simulink model "Human_Driver"  (R2024b)
settings: Solver=ode1  StartTime=0.0  StopTime=inf  FixedStep=0.01  RelTol=1e-3
libraries: rFproPhysicsLib x13
settings Model: ParamWorkspaceSource=ReferencedWorkspace  TunableVars=LOCAL_PORT_RECV,REMOTE_PORT_RECV,gCGHeight,gFrontTrack,gFrontWheelRadius,gLeftWheelBase,gRearTrack,gRearWheelRadius,gRightWheelBase  TunableVarsStorageClass=Auto,Auto,Auto,Auto,Auto,Auto,Auto,Auto,Auto  TunableVarsTypeQualifier=,,,,,,,,  Creator=enewton  LastModifiedBy=Saian
settings SolverCC: AlgebraicLoopSolver=TrustRegion
settings DataIOCC: LimitDataPoints=on  SaveFormat=Array  SignalLoggingSaveFormat=ModelDataLogs  SaveOutput=off  SignalLogging=off  DSMLogging=off  SaveTime=off  ReturnWorkspaceOutputs=off
settings OptimizationCC: BlockReduction=off  ConditionallyExecuteInputs=off  OptimizeBlockIOStorage=off  BufferReuse=off  GlobalBufferReuse=off  ExpressionFolding=off  ExpressionDepthLimit=2147483647  LocalBlockOutputs=off  LifeSpan=inf  OptimizeDataStoreBuffers=off  BusAssignmentInplaceUpdate=off
settings DebuggingCC: UnderspecifiedInitializationDetection=Classic  MergeDetectMultiDrivingBlocksExec=none  SolverPrmCheckMsg=warning  FcnCallInpInsideContextMsg=warning  UnconnectedInputMsg=warning  UnconnectedOutputMsg=warning  UnconnectedLineMsg=warning  StateNameClashWarn=warning  SFUnexpectedBacktrackingDiag=warning  SFNoUnconditionalDefaultTransitionDiag=warning  SFExecutionAtInitializationDiag=none  ArithmeticOperatorsInVariantConditions=warning
settings HardwareCC: ProdBitPerPointer=32  ProdBitPerSizeT=32  ProdBitPerPtrDiffT=32  ProdLargestAtomicFloat=None  ProdIntDivRoundTo=Undefined  ProdEndianess=Unspecified  ProdWordSize=32  ProdHWDeviceType=32-bit Generic
settings ModelReferenceCC: EnableRefExpFcnMdlSchedulingChecks=on  PropagateSignalLabelsOutOfModel=off
settings SFSimCC: SimUseLocalCustomCode=off  CustomCodeUndefinedFunction=UseInterfaceOnly  SimTargetLang=C++
settings RTWCC: Description=rFpro Target (Run Physics)  SystemTargetFile=rfpro.tlc  MakeCommand="make_rtw OPTS=\"-DRUN_PHYSICS\""  TemplateMakefile=rfpro.tmf  RTWUseLocalCustomCode=off  TargetLang=C++  GPUComputeCapability=3.5
settings CodeAppCC: StateflowObjectComments=on
settings STFCustomTargetCC: ModelReferenceCompliant=off  CombineOutputUpdateFcns=on  MatFileLogging=on  CPPClassGenCompliant=on  SystemTargetFile=rfpro.tlc
settings GRTTargetCC: TargetLangStandard=C89/C90 (ANSI)  ModelReferenceCompliant=off  ParMdlRefBuildCompliant=off  CompOptLevelCompliant=off  ConcurrentExecutionCompliant=off  UseToolchainInfoCompliant=off
settings ConfigComp: CovMetricSettings=dw  CovSaveCumulativeToWorkspaceVar=on  CovSaveSingleToWorkspaceVar=on  CovExternalEMLEnable=off

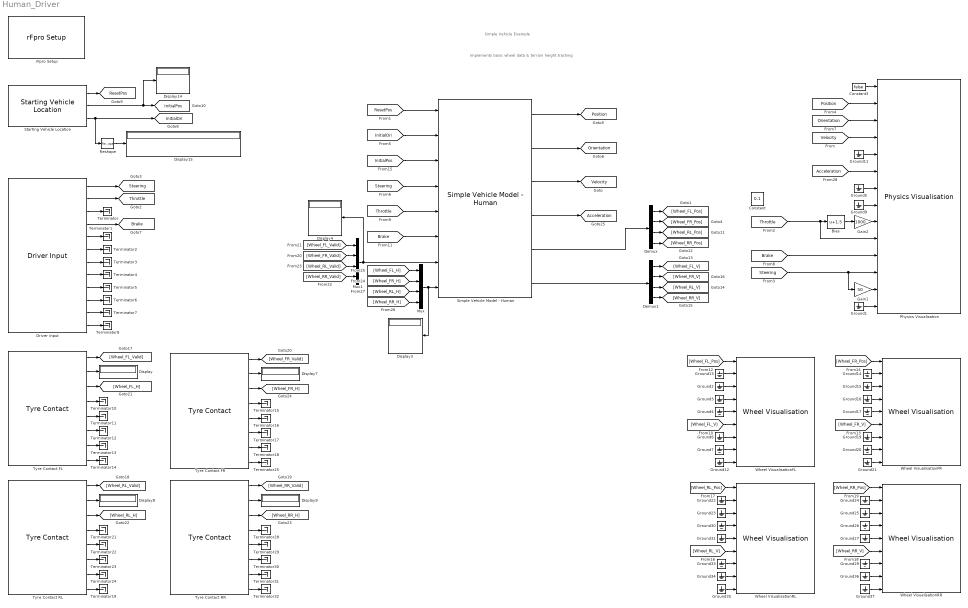
== system Human_Driver ==
  note: Simple Vehicle Example
  note: Implements basic wheel data & terrain height tracking
  Bias : Bias  Bias=1.5  SaturateOnIntegerOverflow=off
  Constant : Constant  Value=0.1
  Constant3 : Constant  Value=false
  Demux : Demux
  Demux1 : Demux
  Display{,3..4,7..9,14..15} (8 alike) : Display
  "Driver Input " : rFproPhysicsLib/Driver Input
      settings: SourceProductName=rFpro Physics
  Gain1 : Gain  Gain=50
  Gain2 : Gain  Gain=1000
  Ground{1..7,9,11..17,19..27,29..31,33..37} (32 alike) : Ground
  Mux : Mux
  Mux1 : Mux
  Physics Visualisation : rFproPhysicsLib/Physics Visualisation  PAR_SKIP_INTERNAL_PHYSICS=off  PAR_ACCEL_VALID=on  PAR_ROT_ACCEL_VALID=off  PAR_GEAR_VALID=off  PAR_RPM_VALID=on  PAR_INPUTS_VALID=on  PAR_STEER_TORQUE_VALID=on  PAR_HEADLIGHTS_ON_VALID=off  PAR_WHEEL_POS_VALID=on  PAR_WHEEL_ORI_VALID=off  PAR_TYRE_PARAMS_VALID=off  PAR_WHEEL_ROTATION_VALID=on  PAR_WHEEL_BRAKE_TEMP_VALID=off  PAR_WHEEL_TREAD_TEMP_VALID=off  PAR_WHEEL_AIR_TEMP_VALID=off  period=-1  offset=0  useReverseByteOrder=on  rFpro__platform=Remote Model - Default
      settings: SourceProductName=rFpro Physics
  Reshape : Reshape  OutputDimensionality=Customize  OutputDimensions=[3,3]
  Simple Vehicle Model - Human : rFproPhysicsLib/Internal Utility/Simple Vehicle Model - Human  TIMESTEP=0.01  gCGHeight=0.52  gLeftWheelBase=4.126  gRightWheelBase=4.126  gFrontTrack=1.55  gRearTrack=1.525  gFrontWheelRadius=0.56  gRearWheelRadius=0.56  gWheelDeflection=0
      link override bConstantSpeed: Value=0
      settings: SourceProductName=rFpro Physics
  Starting Vehicle Location : rFproPhysicsLib/Starting Vehicle Location  cg_offset=CG_OFFSET_FROM_NOSE  numPackets=1  rFpro__platform=Remote Model - Default
      settings: SourceProductName=rFpro Physics
  Terminator{,1..8,10..19,21..25,28..32} (29 alike) : Terminator
  Tyre Contact FL : rFproPhysicsLib/Tyre Contact  LabelModeActiveChoice=rFproLib_RemoteModel  wheel=FL  contact=[]  radius=0.3  width=0.32  sampleTime=0.001  rFpro__platform=Remote Model - Default
      settings: SourceProductName=rFpro Physics
  Tyre Contact FR : rFproPhysicsLib/Tyre Contact  LabelModeActiveChoice=rFproLib_RemoteModel  wheel=FR  contact=[]  radius=0.32  width=0.25  sampleTime=0.001  rFpro__platform=Remote Model - Default
      settings: SourceProductName=rFpro Physics
  Tyre Contact RL : rFproPhysicsLib/Tyre Contact  LabelModeActiveChoice=rFproLib_RemoteModel  wheel=RL  contact=[]  radius=0.33  width=0.25  sampleTime=0.001  rFpro__platform=Remote Model - Default
      settings: SourceProductName=rFpro Physics
  Tyre Contact RR : rFproPhysicsLib/Tyre Contact  LabelModeActiveChoice=rFproLib_RemoteModel  wheel=RR  contact=[]  radius=0.33  width=0.25  sampleTime=0.001  rFpro__platform=Remote Model - Default
      settings: SourceProductName=rFpro Physics
  Wheel VisualisationFL : rFproPhysicsLib/Wheel Visualisation  wheelStr=FL
      settings: SourceProductName=rFpro Physics
  Wheel VisualisationFR : rFproPhysicsLib/Wheel Visualisation  wheelStr=FR
      settings: SourceProductName=rFpro Physics
  Wheel VisualisationRL : rFproPhysicsLib/Wheel Visualisation  wheelStr=RL
      settings: SourceProductName=rFpro Physics
  Wheel VisualisationRR : rFproPhysicsLib/Wheel Visualisation  wheelStr=RR
      settings: SourceProductName=rFpro Physics
  rFpro Setup : rFproPhysicsLib/rFpro Setup  platform=Remote Model - Default  stopOnSessionEnd=on  usePseudoRealtime=on  syncToRF=on  useReverseByteOrder=off  useRfTime=on  minIterations=4  maxIterations=1000  ipReceiveAddress='127.0.0.1'  ipReceivePort=11054  receiveSampleTime=-1  ipTransmitAddress='127.0.0.1'  ipTransmitPort=11052  transmitSampleTime=-1  pluginType=RUN_PHYSICS  sysTarget=xpctarget.tlc  templateMakeFile=xpc_default_tmf  makeCommand=make_rtw  buildDesc=xPC target
      settings: SourceProductName=rFpro Physics
  tag scope: Acceleration=global, Brake=global, InitialOri=global, InitialPos=global, Orientation=global, Position=global, ResetPos=global, Steering=global, Throttle=global, Velocity=global
  wires:
  Starting Vehicle Location/2 -> Display14/1, [InitialPos]
  Constant3/1 -> Physics Visualisation/1
  [Orientation] -> Physics Visualisation/3
  [Position] -> Physics Visualisation/2
  "Driver Input "/3 -> Terminator/1
  "Driver Input "/5 -> Terminator1/1
  "Driver Input "/6 -> Terminator2/1
  "Driver Input "/7 -> Terminator3/1
  "Driver Input "/8 -> Terminator4/1
  "Driver Input "/9 -> Terminator5/1
  "Driver Input "/10 -> Terminator6/1
  "Driver Input "/11 -> Terminator7/1
  "Driver Input "/12 -> Terminator8/1
  [Acceleration] -> Physics Visualisation/6
  Ground9/1 -> Physics Visualisation/8
  Gain2/1 -> Physics Visualisation/9
  Ground11/1 -> Physics Visualisation/5
  Starting Vehicle Location/1 -> [ResetPos]
  Gain1/1 -> Physics Visualisation/13
  Ground1/1 -> Physics Visualisation/14
  Tyre Contact FL/4 -> Terminator10/1
  Tyre Contact FL/5 -> Terminator11/1
  Tyre Contact FL/6 -> Terminator12/1
  Ground2/1 -> Wheel VisualisationFL/3
  Ground3/1 -> Wheel VisualisationFL/4
  Ground4/1 -> Wheel VisualisationFL/5
  Ground6/1 -> Wheel VisualisationFL/7
  Ground7/1 -> Wheel VisualisationFL/8
  Ground12/1 -> Wheel VisualisationFL/9
  Ground13/1 -> Wheel VisualisationFL/2
  Tyre Contact FL/7 -> Terminator13/1
  Tyre Contact FL/2 -> Display/1
  Tyre Contact FL/8 -> Terminator14/1
  Tyre Contact FR/5 -> Terminator16/1
  Tyre Contact FR/6 -> Terminator17/1
  Tyre Contact FR/7 -> Terminator18/1
  Tyre Contact FR/2 -> Display7/1
  Tyre Contact RL/4 -> Terminator21/1
  Tyre Contact RL/5 -> Terminator22/1
  Tyre Contact RL/6 -> Terminator23/1
  Tyre Contact RL/7 -> Terminator24/1
  Tyre Contact RL/2 -> Display8/1
  Tyre Contact RL/8 -> Terminator19/1
  Tyre Contact RR/5 -> Terminator29/1
  Tyre Contact RR/6 -> Terminator30/1
  Tyre Contact RR/7 -> Terminator31/1
  Tyre Contact RR/2 -> Display9/1
  Ground14/1 -> Wheel VisualisationFR/2
  Ground15/1 -> Wheel VisualisationFR/3
  Ground16/1 -> Wheel VisualisationFR/4
  Ground17/1 -> Wheel VisualisationFR/5
  Ground19/1 -> Wheel VisualisationFR/7
  Ground20/1 -> Wheel VisualisationFR/8
  Ground21/1 -> Wheel VisualisationFR/9
  Ground22/1 -> Wheel VisualisationRL/2
  Ground23/1 -> Wheel VisualisationRL/3
  Ground30/1 -> Wheel VisualisationRL/4
  Ground31/1 -> Wheel VisualisationRL/5
  Ground33/1 -> Wheel VisualisationRL/7
  Ground34/1 -> Wheel VisualisationRL/8
  Ground35/1 -> Wheel VisualisationRL/9
  Ground24/1 -> Wheel VisualisationRR/2
  Ground25/1 -> Wheel VisualisationRR/3
  Ground26/1 -> Wheel VisualisationRR/4
  Ground27/1 -> Wheel VisualisationRR/5
  Ground29/1 -> Wheel VisualisationRR/7
  Ground36/1 -> Wheel VisualisationRR/8
  Ground37/1 -> Wheel VisualisationRR/9
  Ground5/1 -> Physics Visualisation/7
  Starting Vehicle Location/3 -> Reshape/1, [InitialOri]
  [InitialOri] -> Simple Vehicle Model - Human/2
  [ResetPos] -> Simple Vehicle Model - Human/1
  [Throttle] -> Simple Vehicle Model - Human/5
  [Brake] -> Simple Vehicle Model - Human/6
  [InitialPos] -> Simple Vehicle Model - Human/3
  [Steering] -> Simple Vehicle Model - Human/4
  Simple Vehicle Model - Human/5 -> Demux/1
  Tyre Contact FR/4 -> Terminator15/1
  Tyre Contact FR/8 -> Terminator25/1
  Simple Vehicle Model - Human/1 -> [Position]
  Simple Vehicle Model - Human/2 -> [Orientation]
  Simple Vehicle Model - Human/3 -> [Velocity]
  Demux/1 -> [Wheel_FL_Pos]
  Demux/2 -> [Wheel_FR_Pos]
  Demux/3 -> [Wheel_RL_Pos]
  Demux/4 -> [Wheel_RR_Pos]
  Demux1/1 -> [Wheel_FL_V]
  Demux1/2 -> [Wheel_FR_V]
  Demux1/3 -> [Wheel_RL_V]
  Demux1/4 -> [Wheel_RR_V]
  Simple Vehicle Model - Human/6 -> Demux1/1
  [Wheel_FL_Pos] -> Wheel VisualisationFL/1
  [Wheel_FL_V] -> Wheel VisualisationFL/6
  [Wheel_FR_Pos] -> Wheel VisualisationFR/1
  [Wheel_FR_V] -> Wheel VisualisationFR/6
  [Wheel_RL_V] -> Wheel VisualisationRL/6
  [Wheel_RL_Pos] -> Wheel VisualisationRL/1
  [Wheel_RR_V] -> Wheel VisualisationRR/6
  [Wheel_RR_Pos] -> Wheel VisualisationRR/1
  Tyre Contact RL/1 -> [Wheel_RL_Valid]
  Tyre Contact RL/3 -> [Wheel_RL_H]
  Tyre Contact RR/1 -> [Wheel_RR_Valid]
  Tyre Contact RR/3 -> [Wheel_RR_H]
  Tyre Contact FR/3 -> [Wheel_FR_H]
  Tyre Contact FR/1 -> [Wheel_FR_Valid]
  Tyre Contact FL/1 -> [Wheel_FL_Valid]
  Tyre Contact FL/3 -> [Wheel_FL_H]
  [Wheel_RL_Valid] -> Mux1/3
  [Wheel_RR_Valid] -> Mux1/4
  [Wheel_FL_Valid] -> Mux1/1
  [Wheel_FR_Valid] -> Mux1/2
  [Wheel_FR_H] -> Mux/2
  [Wheel_FL_H] -> Mux/1
  [Wheel_RR_H] -> Mux/4
  [Wheel_RL_H] -> Mux/3
  Mux1/1 -> Simple Vehicle Model - Human/7, Display4/1
  Mux/1 -> Simple Vehicle Model - Human/8, Display3/1
  Tyre Contact RR/4 -> Terminator28/1
  Tyre Contact RR/8 -> Terminator32/1
  Reshape/1 -> Display15/1
  Bias/1 -> Gain2/1
  Simple Vehicle Model - Human/4 -> [Acceleration]
  "Driver Input "/1 -> [Steering]
  "Driver Input "/2 -> [Throttle]
  "Driver Input "/4 -> [Brake]
  [Brake] -> Physics Visualisation/11
  [Steering] -> Gain1/1, Physics Visualisation/12
  [Velocity] -> Physics Visualisation/4
  [Throttle] -> Physics Visualisation/10, Bias/1
